simulink model "MLC_Aero_Simulink"  (R2021b)
settings: Solver=ode1  StartTime=0.0  StopTime=inf  FixedStep=0.002  RelTol=1e-3  EnableMultiTasking=on
undefined symbols (not defined in the file): HIL, qc_get_step_size
libraries: quarc_library x6, cstblocks x5
settings Model: SimulationMode=external  ExtModeTrigDuration=20000  Creator=MLevis  LastModifiedBy=hongp
settings SolverCC: AlgebraicLoopSolver=TrustRegion  PositivePriorityOrder=on
settings DataIOCC: LimitDataPoints=on  SaveFormat=Array  ReturnWorkspaceOutputs=off
settings OptimizationCC: LifeSpan=inf
settings DebuggingCC: SolverPrmCheckMsg=warning  SFUnexpectedBacktrackingDiag=warning  SFNoUnconditionalDefaultTransitionDiag=warning  SFExecutionAtInitializationDiag=none  SFMachineParentedDataDiag=warning  ArithmeticOperatorsInVariantConditions=warning
settings HardwareCC: ProdBitPerPointer=32  ProdBitPerSizeT=32  ProdBitPerPtrDiffT=32  ProdLargestAtomicFloat=None  ProdIntDivRoundTo=Undefined  ProdEndianess=Unspecified  ProdWordSize=32  ProdHWDeviceType=32-bit Generic
settings ModelReferenceCC: PropagateSignalLabelsOutOfModel=off
settings SFSimCC: SimUseLocalCustomCode=off  CustomCodeUndefinedFunction=UseInterfaceOnly
settings RTWCC: Description=QUARC Win64 Target  SystemTargetFile=quarc_win64.tlc  TemplateMakefile=quarc_default_tmf  RTWUseLocalCustomCode=off
settings CodeAppCC: StateflowObjectComments=on
settings STFCustomTargetCC: TargetPreCompLibLocation=C:\PROGRA~3\QUARC\lib\2016a\win64\release  ConcurrentExecutionCompliant=on  SystemTargetFile=quarc_win64.tlc
settings GRTTargetCC: TargetPreCompLibLocation=C:\PROGRA~3\QUARC\lib\2016a\win64\release  TargetLangStandard=C89/C90 (ANSI)  ParMdlRefBuildCompliant=off  CompOptLevelCompliant=off  CombineOutputUpdateFcns=off  MatFileLogging=off  CPPClassGenCompliant=off  GRTInterface=on  UseToolchainInfoCompliant=off  ExtMode=on  ExtModeMexFile=quarc_comm
settings ConfigComp: CovMetricSettings=dw  CovSaveCumulativeToWorkspaceVar=on  CovSaveSingleToWorkspaceVar=on  CovExternalEMLEnable=off  CovSFcnEnable=off

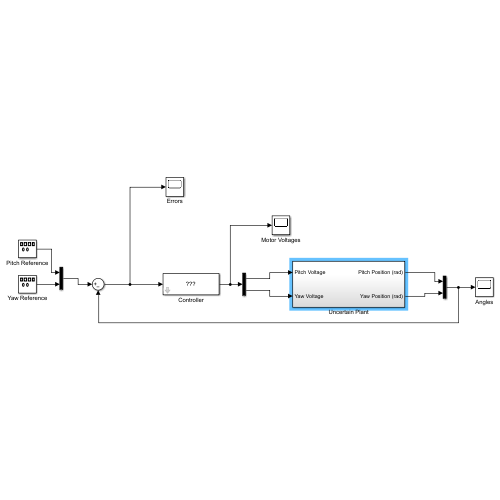
[thumbnail: Simulink's stored preview of the top-level diagram]
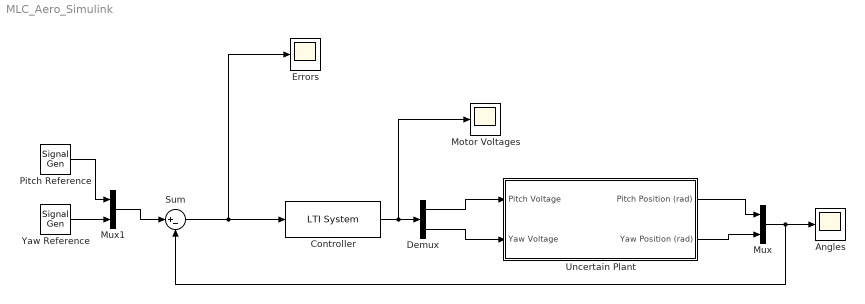
== system MLC_Aero_Simulink ==
  Angles : Scope
  Controller : cstblocks/LTI System  sys=K  IC=[]
  Demux : Demux  Outputs=2
  Errors : Scope
  Motor Voltages : Scope
  Mux : Mux  Inputs=2
  Mux1 : Mux  Inputs=2
  "Pitch Reference " : SignalGenerator  WaveForm=square  Amplitude=pi/6  Frequency=0.4  Units=rad/sec
  Sum : Sum  Inputs=|+-
  Uncertain Plant : Subsystem
  Yaw Reference : SignalGenerator  Amplitude=pi/4  Frequency=0.5  Units=rad/sec
  wires:
  Controller/1 -> Motor Voltages/1, Demux/1
  Demux/1 -> Uncertain Plant/1(Pitch Voltage)
  Demux/2 -> Uncertain Plant/2(Yaw Voltage)
  Sum/1 -> Errors/1, Controller/1
  Uncertain Plant/1(Pitch Position (rad)) -> Mux/1
  Uncertain Plant/2(Yaw Position (rad)) -> Mux/2
  Mux/1 -> Sum/2, Angles/1
  "Pitch Reference "/1 -> Mux1/1
  Yaw Reference/1 -> Mux1/2
  Mux1/1 -> Sum/1

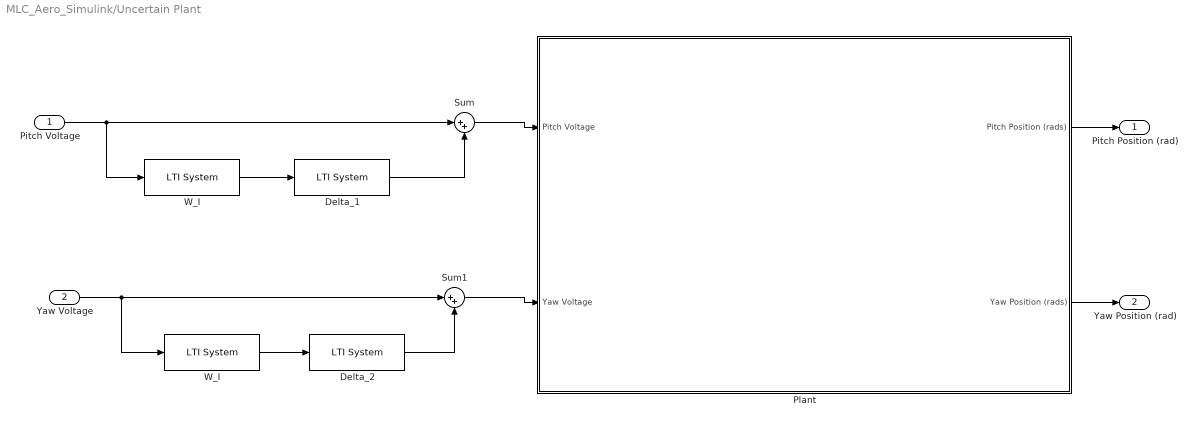
== system MLC_Aero_Simulink/Uncertain Plant ==
  Pitch Voltage : Inport
  Yaw Voltage : Inport  Port=2
  Delta_1 : cstblocks/LTI System  sys=Delta_1  IC=[]
  Delta_2 : cstblocks/LTI System  sys=Delta_2  IC=[]
  Plant : Subsystem
  Sum : Sum  Inputs=|++
  Sum1 : Sum  Inputs=|++
  W_I : cstblocks/LTI System  sys=W_I_Pitch  IC=[]
  "W_I " : cstblocks/LTI System  sys=W_I_Yaw  IC=[]
  Pitch Position (rad) : Outport
  Yaw Position (rad) : Outport  Port=2
  wires:
  W_I/1 -> Delta_1/1
  Sum/1 -> Plant/1(Pitch Voltage)
  Pitch Voltage/1 -> W_I/1, Sum/1
  Delta_1/1 -> Sum/2
  Sum1/1 -> Plant/2(Yaw Voltage)
  Yaw Voltage/1 -> "W_I "/1, Sum1/1
  Delta_2/1 -> Sum1/2
  "W_I "/1 -> Delta_2/1
  Plant/1(Pitch Position (rads)) -> Pitch Position (rad)/1
  Plant/2(Yaw Position (rads)) -> Yaw Position (rad)/1

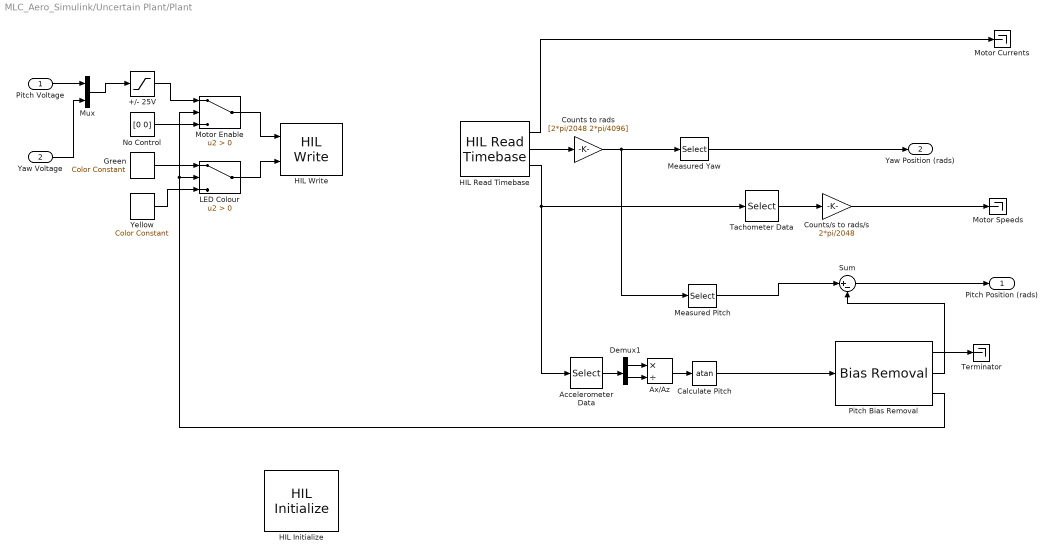
== system MLC_Aero_Simulink/Uncertain Plant/Plant ==
  Pitch Voltage : Inport
  Yaw Voltage : Inport  Port=2
  +/- 25V : Saturate  UpperLimit=25  LowerLimit=-25
  Accelerometer Data : Selector  InputPortWidth=4  IndexOptions=Index vector (dialog)  Indices=[1 2]  OutputSizes=1
  Ax/Az : Product  Inputs=*/
  Calculate Pitch : Trigonometry  Operator=atan
  Counts to rads : Gain  Gain=[2*pi/2048 2*pi/4096]
  Counts/s to rads/s : Gain  Gain=2*pi/2048
  Demux1 : Demux  Outputs=2
  Green : quarc_library/Sources/Signals/Color Constant  color=[0 1 0]
  HIL Initialize : quarc_library/Data Acquisition/Generic/Configuration/HIL Initialize  Priority=-99  object_name=HIL-1  board_type=quanser_aero_usb  board_number=0  board_options=""  exclusive=off  active=off  hardware_clocks=[0]  clock_modes=[]  initial_clock_frequencies=[]  set_clock_params_at_start=off  set_clock_params_at_switch_in=off  set_clock_frequencies_at_start=off  set_clock_frequencies_at_switch_in=off  analog_input_channels=[0:1]  analog_input_configurations=0  analog_input_maximums=3  analog_input_minimums=-3  set_analog_input_params_at_start=off  set_analog_input_params_at_switch_in=off  analog_output_channels=[0:1]  analog_output_maximums=24  analog_output_minimums=-24  initial_analog_outputs=[0]  final_analog_outputs=[0]  watchdog_analog_outputs=[0]  set_analog_output_params_at_start=off  set_analog_output_params_at_switch_in=off  set_analog_outputs_at_start=on  set_analog_outputs_at_switch_in=off  set_analog_outputs_at_terminate=on  set_analog_outputs_at_switch_out=off  set_analog_outputs_on_watchdog=on  digital_input_channels=[]  digital_output_channels=[0:1]  digital_output_configuration=[]  initial_digital_outputs=[1]  final_digital_outputs=[0]  watchdog_digital_outputs=[0]  set_digital_output_params_at_start=off  set_digital_output_params_at_switch_in=off  set_digital_outputs_at_start=on  set_digital_outputs_at_switch_in=off  set_digital_outputs_at_terminate=on  set_digital_outputs_at_switch_out=off  set_digital_outputs_on_watchdog=on  encoder_channels=[0:3]  quadrature=[4]  encoder_filter_frequency=[]  initial_encoder_counts=[0]  set_encoder_params_at_start=off  set_encoder_params_at_switch_in=off  set_encoder_counts_at_start=on  set_encoder_counts_at_switch_in=off  pwm_channels=[]  pwm_modes=[]  pwm_frequency=[]  pwm_configuration=[]  pwm_alignment=[]  pwm_polarity=[]  pwm_leading_deadband=[]  pwm_trailing_deadband=[]  initial_pwm_outputs=[]  final_pwm_outputs=[]  watchdog_pwm_outputs=[]  set_pwm_params_at_start=off  set_pwm_params_at_switch_in=off  set_pwm_outputs_at_start=off  set_pwm_outputs_at_switch_in=off  set_pwm_outputs_at_terminate=off  set_pwm_outputs_at_switch_out=off  set_pwm_outputs_on_watchdog=off  other_output_channels=[11000:11002]  initial_other_outputs=[0 1 0]  final_other_outputs=[1 0 0]  watchdog_other_outputs=[0 0 1]  set_other_outputs_at_start=on  set_other_outputs_at_switch_in=off  set_other_outputs_at_terminate=on  set_other_outputs_at_switch_out=off  set_other_outputs_on_watchdog=on
  HIL Read Timebase : quarc_library/Data Acquisition/Generic/Timebases/HIL Read Timebase  object_name=HIL-1  clock=0  analog_channels=[0:1]  encoder_channels=[2:3]  digital_channels=[]  other_channels=[4000 4002 14000 14001]  samples_in_buffer=max(ceil(1/qc_get_step_size), 1)  active=on  vector_output=on  data_type_mode=Inherit via back propagation  encoder_data_type=double  digital_data_type=boolean
  HIL Write : quarc_library/Data Acquisition/Generic/Immediate I//O/HIL Write  object_name=HIL-1  analog_channels=[0:1]  pwm_channels=[]  digital_channels=[]  other_channels=[11000:11002]  sample_time=-1  active=off  vector_input=on
  LED Colour : Switch  Criteria=u2 > Threshold
  Measured Pitch : Selector  InputPortWidth=2  IndexOptions=Index vector (dialog)  Indices=[1]  OutputSizes=1
  Measured Yaw : Selector  InputPortWidth=2  IndexOptions=Index vector (dialog)  Indices=[2]  OutputSizes=1
  Motor Currents : Terminator
  Motor Enable : Switch  Criteria=u2 > Threshold
  Motor Speeds : Terminator
  Mux : Mux  Inputs=2
  No Control : Constant  Value=[0 0]
  Pitch Bias Removal : quarc_library/Discrete/Bias Removal  start_time=0  end_time=1  switch_id=0  sample_time=qc_get_step_size
  Sum : Sum  Inputs=|+-
  Tachometer Data : Selector  InputPortWidth=4  IndexOptions=Index vector (dialog)  Indices=[3 4]  OutputSizes=1
  Terminator : Terminator
  Yellow : quarc_library/Sources/Signals/Color Constant  color=[1 1 0]
  Pitch Position (rads) : Outport
  Yaw Position (rads) : Outport  Port=2
  wires:
  Pitch Bias Removal/3 -> Motor Enable/2, LED Colour/2
  +/- 25V/1 -> Motor Enable/1
  Motor Enable/1 -> HIL Write/1
  Green/1 -> LED Colour/1
  Yellow/1 -> LED Colour/3
  LED Colour/1 -> HIL Write/2
  No Control/1 -> Motor Enable/3
  Tachometer Data/1 -> Counts/s to rads/s/1
  Demux1/1 -> Ax/Az/1
  Demux1/2 -> Ax/Az/2
  HIL Read Timebase/2 -> Counts to rads/1
  Calculate Pitch/1 -> Pitch Bias Removal/1
  Counts/s to rads/s/1 -> Motor Speeds/1
  HIL Read Timebase/1 -> Motor Currents/1
  Accelerometer Data/1 -> Demux1/1
  HIL Read Timebase/3 -> Accelerometer Data/1, Tachometer Data/1
  Counts to rads/1 -> Measured Pitch/1, Measured Yaw/1
  Ax/Az/1 -> Calculate Pitch/1
  Pitch Bias Removal/2 -> Sum/2
  Pitch Voltage/1 -> Mux/1
  Yaw Voltage/1 -> Mux/2
  Mux/1 -> +/- 25V/1
  Pitch Bias Removal/1 -> Terminator/1
  Sum/1 -> Pitch Position (rads)/1
  Measured Pitch/1 -> Sum/1
  Measured Yaw/1 -> Yaw Position (rads)/1
